simulink model "pmsm_with_saliency_and_damper"  (R2020a)
settings: Solver=FixedStepAuto  StartTime=0.0  StopTime=5  RelTol=1e-3  AbsTol=0.1
InitFcn:
  | vm=400;
  | wbase=314;
  | f=50;
  | xls=0.00291*wbase;
  | rs=0.037;
  | xmq=0.00324*wbase;
  | xmd=0.00324*wbase;
  | rkq=0.00144;
  | xlkq=0.6578;
  | rkd=0.1080;
  | xlkd=0.06577;
  | xaq=((1/xmq)+(1/xls)+(1/xlkq))^-1;
  | xad=((1/xmd)+(1/xls)+(1/xlkd))^-1;
  | Tl=50;
  | lamda_magnet=0.162;
  | p=10;
  | b=5*10^-3;
  | j=0.0003;
model workspace (MAT data in the model file):
  wb = Simulink.Parameter
  wb.DataType = 'auto'
  wb.Dimensions = [0 0]
settings Model: SnapshotBufferSize=100  SnapshotInterval=100  Creator=moham  LastModifiedBy=moham
settings SolverCC: ZeroCrossControl=EnableAll  AlgebraicLoopSolver=LineSearch
settings OptimizationCC: OptimizeBlockIOStorage=off  OptimizeDataStoreBuffers=off  BusAssignmentInplaceUpdate=off
settings DebuggingCC: SFUnexpectedBacktrackingDiag=warning  SFNoUnconditionalDefaultTransitionDiag=warning
settings RTWCC: Description=Generic Real-Time Target  GenCodeOnly=on  GenerateReport=on  BuildConfiguration=Debug  LaunchReport=on  RTWCompilerOptimization=on
settings CodeAppCC: ForceParamTrailComments=on  MaxIdLength=95  MATLABSourceComments=on  EnableCustomComments=on
settings GRTTargetCC: CombineSignalStateStructs=on  SupportVariableSizeSignals=on  MultiInstanceErrorCode=Warning

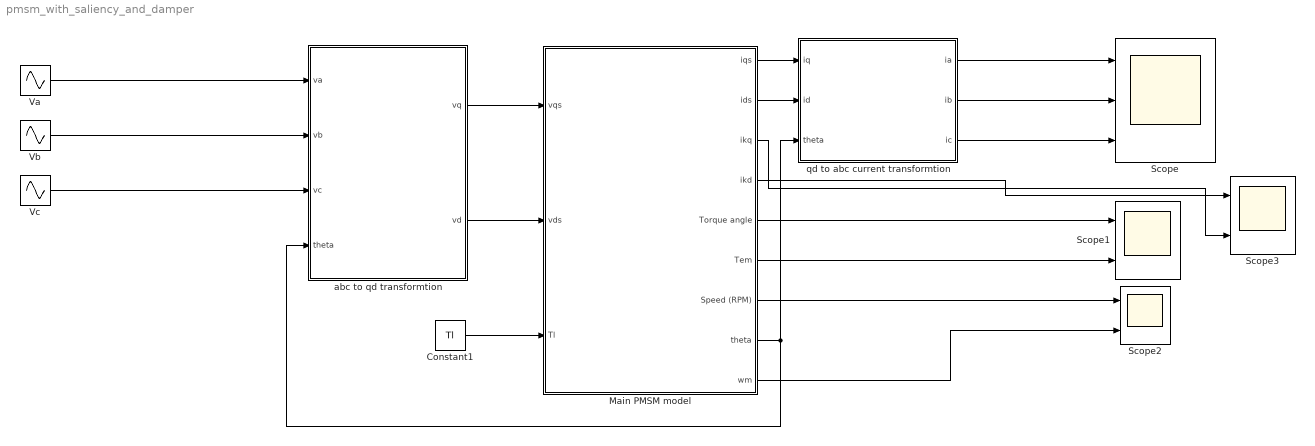
== system pmsm_with_saliency_and_damper ==
  Constant1 : Constant  Value=Tl
  Main PMSM model : Subsystem
  Scope : Scope  NumInputPorts=3
  Scope1 : Scope  NumInputPorts=2
  Scope2 : Scope  NumInputPorts=2
  Scope3 : Scope  NumInputPorts=2
  Va : Sin  Amplitude=vm  Frequency=2*pi*f  SampleTime=0.0001
  Vb : Sin  Amplitude=vm  Frequency=2*pi*f  Phase=-(2*pi/3)  SampleTime=0.0001
  Vc : Sin  Amplitude=vm  Frequency=2*pi*f  Phase=2*pi/3  SampleTime=0.0001
  abc to qd transformtion : Subsystem
  qd to abc current transformtion : Subsystem
  wires:
  Main PMSM model/2(ids) -> qd to abc current transformtion/2(id)
  Main PMSM model/8("theta ") -> abc to qd transformtion/4(theta), qd to abc current transformtion/3(theta)
  abc to qd transformtion/2(vd) -> Main PMSM model/2(vds)
  Constant1/1 -> Main PMSM model/3(Tl)
  abc to qd transformtion/1(vq) -> Main PMSM model/1(vqs)
  Main PMSM model/1(iqs) -> qd to abc current transformtion/1(iq)
  Va/1 -> abc to qd transformtion/1(va)
  Vb/1 -> abc to qd transformtion/2(vb)
  Vc/1 -> abc to qd transformtion/3(vc)
  qd to abc current transformtion/1(ia) -> Scope/1
  qd to abc current transformtion/2(ib) -> Scope/2
  qd to abc current transformtion/3(ic) -> Scope/3
  Main PMSM model/5(Torque angle) -> Scope1/1
  Main PMSM model/6(Tem) -> Scope1/2
  Main PMSM model/7(Speed (RPM)) -> Scope2/1
  Main PMSM model/9(wm) -> Scope2/2
  Main PMSM model/4(ikd) -> Scope3/1
  Main PMSM model/3(ikq) -> Scope3/2

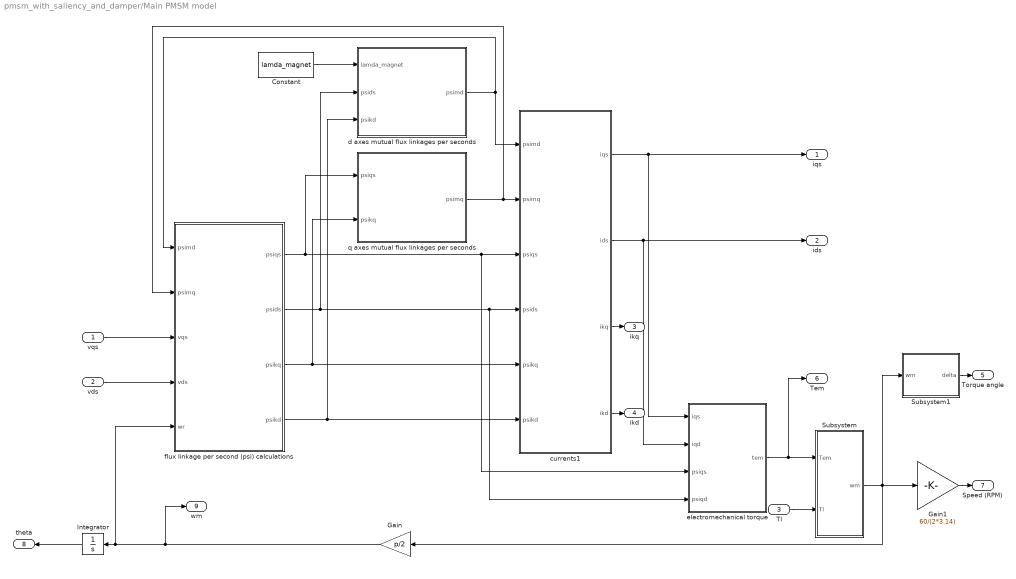
== system pmsm_with_saliency_and_damper/Main PMSM model ==
  vqs : Inport
  vds : Inport  Port=2
  Tl : Inport  Port=3
  Constant : Constant  Value=lamda_magnet
  Gain : Gain  Gain=p/2
  Gain1 : Gain  Gain=60/(2*3.14)
  Integrator : Integrator
  Subsystem : Subsystem
  Subsystem1 : Subsystem
  currents1 : Subsystem
  d axes mutual flux linkages per seconds : Subsystem
  electromechanical torque : Subsystem
  flux linkage per second (psi) calculations : Subsystem
  q axes mutual flux linkages per seconds : Subsystem
  iqs : Outport
  ids : Outport  Port=2
  ikq : Outport  Port=3
  ikd : Outport  Port=4
  Torque angle : Outport  Port=5
  Tem : Outport  Port=6
  Speed (RPM) : Outport  Port=7
  "theta " : Outport  Port=8
  wm : Outport  Port=9
  wires:
  currents1/2(ids) -> ids/1, electromechanical torque/2(iqd)
  q axes mutual flux linkages per seconds/1(psimq) -> flux linkage per second (psi) calculations/2(psimq), currents1/2(psimq)
  flux linkage per second (psi) calculations/2(psids) -> d axes mutual flux linkages per seconds/2(psids), currents1/4(psids), electromechanical torque/4(psiqd)
  electromechanical torque/1(tem) -> Tem/1, Subsystem/1(Tem)
  d axes mutual flux linkages per seconds/1(psimd) -> flux linkage per second (psi) calculations/1(psimd), currents1/1(psimd)
  currents1/1(iqs) -> iqs/1, electromechanical torque/1(iqs)
  currents1/4(ikd) -> ikd/1
  currents1/3(ikq) -> ikq/1
  Gain/1 -> wm/1, flux linkage per second (psi) calculations/5(wr), Integrator/1
  Constant/1 -> d axes mutual flux linkages per seconds/1(lamda_magnet)
  Subsystem/1(wm) -> Gain/1, Gain1/1, Subsystem1/1(wm)
  flux linkage per second (psi) calculations/3(psikq) -> q axes mutual flux linkages per seconds/2(psikq), currents1/5(psikq)
  flux linkage per second (psi) calculations/4(psikd) -> d axes mutual flux linkages per seconds/3(psikd), currents1/6(psikd)
  flux linkage per second (psi) calculations/1(psiqs) -> q axes mutual flux linkages per seconds/1(psiqs), currents1/3(psiqs), electromechanical torque/3(psiqs)
  vqs/1 -> flux linkage per second (psi) calculations/3(vqs)
  Gain1/1 -> Speed (RPM)/1
  vds/1 -> flux linkage per second (psi) calculations/4(vds)
  Subsystem1/1(delta) -> Torque angle/1
  Tl/1 -> Subsystem/2(Tl)
  Integrator/1 -> "theta "/1

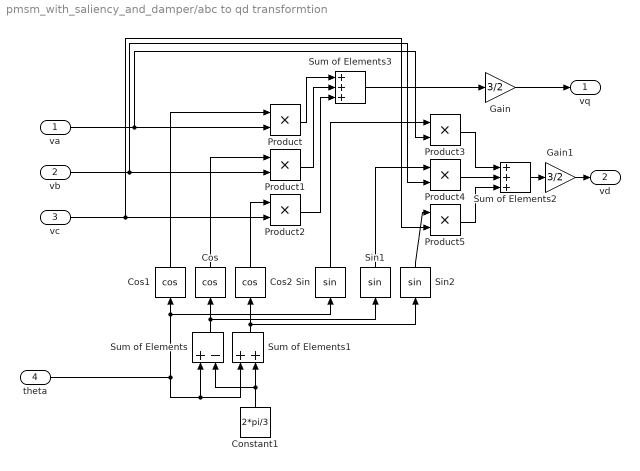
== system pmsm_with_saliency_and_damper/abc to qd transformtion ==
  va : Inport
  vb : Inport  Port=2
  vc : Inport  Port=3
  theta : Inport  Port=4
  Constant1 : Constant  Value=2*pi/3
  Cos : Trigonometry  Operator=cos
  Cos1 : Trigonometry  Operator=cos
  Cos2 : Trigonometry  Operator=cos
  Gain : Gain  Gain=3/2
  Gain1 : Gain  Gain=3/2
  Product{,1..5} (6 alike) : Product
  Sin : Trigonometry
  Sin1 : Trigonometry
  Sin2 : Trigonometry
  Sum of Elements : Sum  Inputs=+-
  Sum of Elements1 : Sum
  Sum of Elements2 : Sum  Inputs=+++
  Sum of Elements3 : Sum  Inputs=+++
  vq : Outport
  vd : Outport  Port=2
  wires:
  vc/1 -> Product2/2, Product5/2
  theta/1 -> Sum of Elements1/1, Sum of Elements/1, Sin/1, Cos1/1
  va/1 -> Product3/2, Product/2
  vb/1 -> Product1/2, Product4/2
  Cos/1 -> Product1/1
  Constant1/1 -> Sum of Elements1/2, Sum of Elements/2
  Cos1/1 -> Product/1
  Product/1 -> Sum of Elements3/1
  Sin/1 -> Product3/1
  Product1/1 -> Sum of Elements3/2
  Sum of Elements/1 -> Sin1/1, Cos/1
  Sin2/1 -> Product5/1
  Product5/1 -> Sum of Elements2/3
  Sum of Elements3/1 -> Gain/1
  Sum of Elements1/1 -> Sin2/1, Cos2/1
  Product3/1 -> Sum of Elements2/1
  Product4/1 -> Sum of Elements2/2
  Product2/1 -> Sum of Elements3/3
  Cos2/1 -> Product2/1
  Sin1/1 -> Product4/1
  Gain/1 -> vq/1
  Gain1/1 -> vd/1
  Sum of Elements2/1 -> Gain1/1

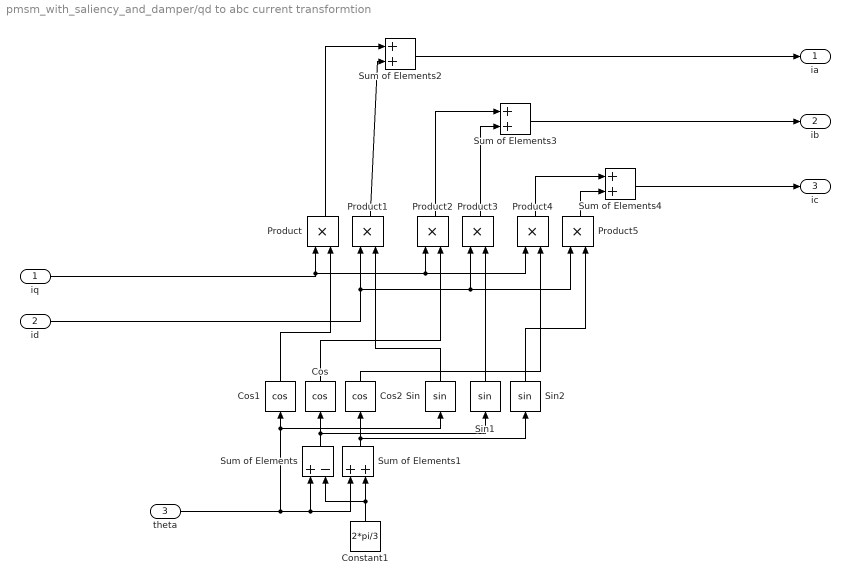
== system pmsm_with_saliency_and_damper/qd to abc current transformtion ==
  iq : Inport
  id : Inport  Port=2
  theta : Inport  Port=3
  Constant1 : Constant  Value=2*pi/3
  Cos : Trigonometry  Operator=cos
  Cos1 : Trigonometry  Operator=cos
  Cos2 : Trigonometry  Operator=cos
  Product{,1..5} (6 alike) : Product
  Sin : Trigonometry
  Sin1 : Trigonometry
  Sin2 : Trigonometry
  Sum of Elements : Sum  Inputs=+-
  Sum of Elements{1..4} (4 alike) : Sum
  ia : Outport
  ib : Outport  Port=2
  ic : Outport  Port=3
  wires:
  theta/1 -> Sin/1, Cos1/1, Sum of Elements1/1, Sum of Elements/1
  Constant1/1 -> Sum of Elements1/2, Sum of Elements/2
  Sum of Elements/1 -> Sin1/1, Cos/1
  Sum of Elements1/1 -> Sin2/1, Cos2/1
  iq/1 -> Product2/1, Product4/1, Product/1
  Cos1/1 -> Product/2
  id/1 -> Product1/1, Product3/1, Product5/1
  Sin/1 -> Product1/2
  Cos/1 -> Product2/2
  Sin1/1 -> Product3/2
  Cos2/1 -> Product4/2
  Sin2/1 -> Product5/2
  Product1/1 -> Sum of Elements2/2
  Product/1 -> Sum of Elements2/1
  Product3/1 -> Sum of Elements3/2
  Product2/1 -> Sum of Elements3/1
  Product5/1 -> Sum of Elements4/2
  Product4/1 -> Sum of Elements4/1
  Sum of Elements2/1 -> ia/1
  Sum of Elements3/1 -> ib/1
  Sum of Elements4/1 -> ic/1

== system pmsm_with_saliency_and_damper/Main PMSM model/Subsystem ==
  Tem : Inport
  Tl : Inport  Port=2
  Constant2 : Constant  Value=b
  Constant3 : Constant  Value=j
  Divide : Product  Inputs=*/
  Integrator1 : Integrator
  Product2 : Product
  Sum of Elements1 : Sum  Inputs=+--
  wm : Outport
  wires:
  Tem/1 -> Sum of Elements1/1
  Sum of Elements1/1 -> Divide/1
  Constant3/1 -> Divide/2
  Product2/1 -> Sum of Elements1/3
  Divide/1 -> Integrator1/1
  Integrator1/1 -> wm/1, Product2/1
  Tl/1 -> Sum of Elements1/2
  Constant2/1 -> Product2/2

== system pmsm_with_saliency_and_damper/Main PMSM model/Subsystem1 ==
  wm : Inport
  Constant : Constant  Value=p/2
  Constant2 : Constant  Value=2*pi*f
  Integrator1 : Integrator
  Product : Product
  Sum of Elements : Sum  Inputs=+-
  delta : Outport
  wires:
  Sum of Elements/1 -> Integrator1/1
  Integrator1/1 -> delta/1
  Constant2/1 -> Sum of Elements/1
  wm/1 -> Product/1
  Product/1 -> Sum of Elements/2
  Constant/1 -> Product/2

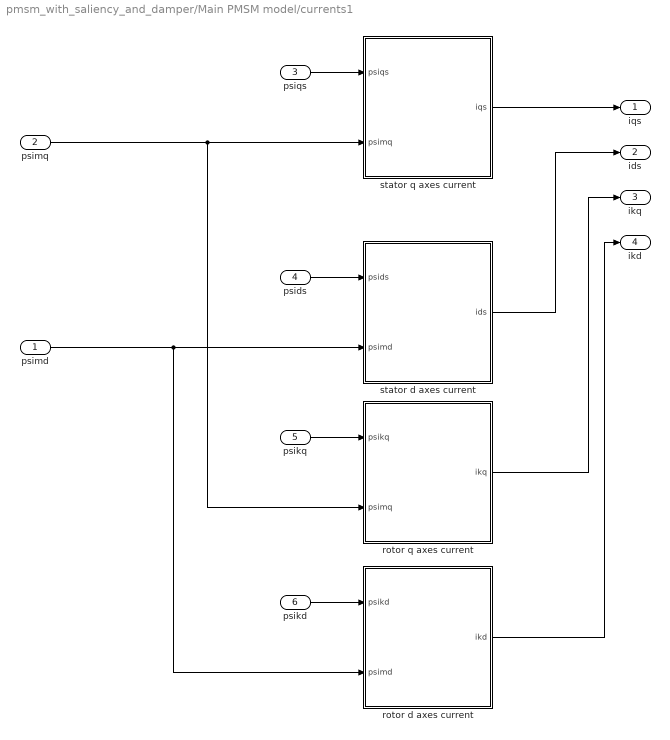
== system pmsm_with_saliency_and_damper/Main PMSM model/currents1 ==
  psimd : Inport
  psimq : Inport  Port=2
  psiqs : Inport  Port=3
  psids : Inport  Port=4
  psikq : Inport  Port=5
  psikd : Inport  Port=6
  rotor d axes current : Subsystem
  rotor q axes current : Subsystem
  stator d axes current : Subsystem
  stator q axes current : Subsystem
  iqs : Outport
  ids : Outport  Port=2
  ikq : Outport  Port=3
  ikd : Outport  Port=4
  wires:
  rotor q axes current/1(ikq) -> ikq/1
  stator q axes current/1(iqs) -> iqs/1
  psikd/1 -> rotor d axes current/1(psikd)
  psids/1 -> stator d axes current/1(psids)
  psimd/1 -> rotor d axes current/2(psimd), stator d axes current/2(psimd)
  stator d axes current/1(ids) -> ids/1
  psimq/1 -> stator q axes current/2(psimq), rotor q axes current/2(psimq)
  rotor d axes current/1(ikd) -> ikd/1
  psikq/1 -> rotor q axes current/1(psikq)
  psiqs/1 -> stator q axes current/1(psiqs)

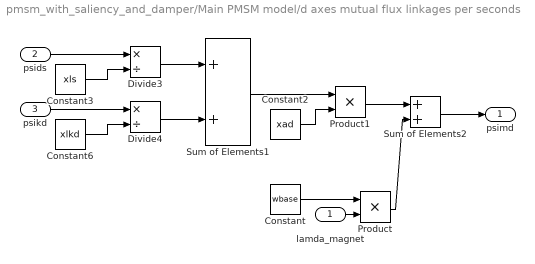
== system pmsm_with_saliency_and_damper/Main PMSM model/d axes mutual flux linkages per seconds ==
  lamda_magnet : Inport
  psids : Inport  Port=2
  psikd : Inport  Port=3
  Constant : Constant  Value=wbase
  Constant2 : Constant  Value=xad
  Constant3 : Constant  Value=xls
  Constant6 : Constant  Value=xlkd
  Divide3 : Product  Inputs=*/
  Divide4 : Product  Inputs=*/
  Product : Product
  Product1 : Product
  Sum of Elements1 : Sum
  Sum of Elements2 : Sum
  psimd : Outport
  wires:
  lamda_magnet/1 -> Product/2
  Sum of Elements1/1 -> Product1/1
  Constant/1 -> Product/1
  Product1/1 -> Sum of Elements2/1
  Constant2/1 -> Product1/2
  Sum of Elements2/1 -> psimd/1
  Product/1 -> Sum of Elements2/2
  psids/1 -> Divide3/1
  psikd/1 -> Divide4/1
  Constant3/1 -> Divide3/2
  Constant6/1 -> Divide4/2
  Divide3/1 -> Sum of Elements1/1
  Divide4/1 -> Sum of Elements1/2

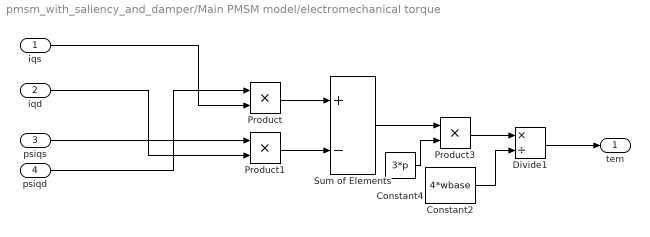
== system pmsm_with_saliency_and_damper/Main PMSM model/electromechanical torque ==
  iqs : Inport
  iqd : Inport  Port=2
  psiqs : Inport  Port=3
  psiqd : Inport  Port=4
  Constant2 : Constant  Value=4*wbase
  Constant4 : Constant  Value=3*p
  Divide1 : Product  Inputs=*/
  Product : Product
  Product1 : Product
  Product3 : Product
  Sum of Elements : Sum  Inputs=+-
  tem : Outport
  wires:
  iqs/1 -> Product/2
  Product1/1 -> Sum of Elements/2
  Product/1 -> Sum of Elements/1
  Sum of Elements/1 -> Product3/1
  psiqs/1 -> Product1/1
  psiqd/1 -> Product/1
  iqd/1 -> Product1/2
  Constant4/1 -> Product3/2
  Constant2/1 -> Divide1/2
  Product3/1 -> Divide1/1
  Divide1/1 -> tem/1

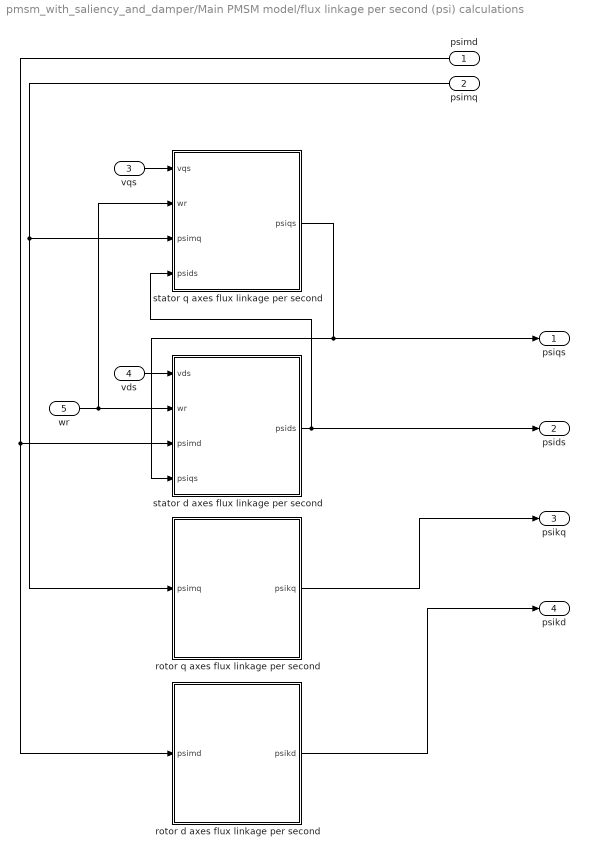
== system pmsm_with_saliency_and_damper/Main PMSM model/flux linkage per second (psi) calculations ==
  psimd : Inport
  psimq : Inport  Port=2
  vqs : Inport  Port=3
  vds : Inport  Port=4
  wr : Inport  Port=5
  rotor d axes flux linkage per second : Subsystem
  rotor q axes flux linkage per second : Subsystem
  stator d axes flux linkage per second : Subsystem
  stator q axes flux linkage per second : Subsystem
  psiqs : Outport
  psids : Outport  Port=2
  psikq : Outport  Port=3
  psikd : Outport  Port=4
  wires:
  stator q axes flux linkage per second/1(psiqs) -> psiqs/1, stator d axes flux linkage per second/4(psiqs)
  rotor q axes flux linkage per second/1(psikq) -> psikq/1
  wr/1 -> stator q axes flux linkage per second/2(wr), stator d axes flux linkage per second/2(wr)
  stator d axes flux linkage per second/1(psids) -> psids/1, stator q axes flux linkage per second/4(psids)
  psimq/1 -> stator q axes flux linkage per second/3(psimq), rotor q axes flux linkage per second/1(psimq)
  vqs/1 -> stator q axes flux linkage per second/1(vqs)
  rotor d axes flux linkage per second/1(psikd) -> psikd/1
  psimd/1 -> rotor d axes flux linkage per second/1(psimd), stator d axes flux linkage per second/3(psimd)
  vds/1 -> stator d axes flux linkage per second/1(vds)

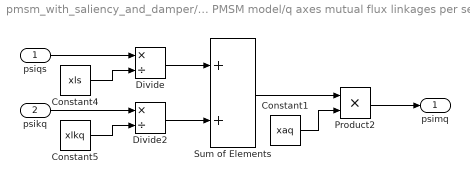
== system pmsm_with_saliency_and_damper/Main PMSM model/q axes mutual flux linkages per seconds ==
  psiqs : Inport
  psikq : Inport  Port=2
  Constant1 : Constant  Value=xaq
  Constant4 : Constant  Value=xls
  Constant5 : Constant  Value=xlkq
  Divide : Product  Inputs=*/
  Divide2 : Product  Inputs=*/
  Product2 : Product
  Sum of Elements : Sum
  psimq : Outport
  wires:
  Divide2/1 -> Sum of Elements/2
  Constant1/1 -> Product2/2
  Constant5/1 -> Divide2/2
  psikq/1 -> Divide2/1
  psiqs/1 -> Divide/1
  Divide/1 -> Sum of Elements/1
  Product2/1 -> psimq/1
  Sum of Elements/1 -> Product2/1
  Constant4/1 -> Divide/2

== system pmsm_with_saliency_and_damper/Main PMSM model/currents1/rotor d axes current ==
  psikd : Inport
  psimd : Inport  Port=2
  Constant : Constant  Value=xlkd
  Divide : Product  Inputs=*/
  Sum of Elements : Sum  Inputs=+-
  ikd : Outport
  wires:
  Divide/1 -> ikd/1
  Constant/1 -> Divide/2
  Sum of Elements/1 -> Divide/1
  psimd/1 -> Sum of Elements/2
  psikd/1 -> Sum of Elements/1

== system pmsm_with_saliency_and_damper/Main PMSM model/currents1/rotor q axes current ==
  psikq : Inport
  psimq : Inport  Port=2
  Constant : Constant  Value=xlkq
  Divide : Product  Inputs=*/
  Sum of Elements : Sum  Inputs=+-
  ikq : Outport
  wires:
  Divide/1 -> ikq/1
  Constant/1 -> Divide/2
  Sum of Elements/1 -> Divide/1
  psimq/1 -> Sum of Elements/2
  psikq/1 -> Sum of Elements/1

== system pmsm_with_saliency_and_damper/Main PMSM model/currents1/stator d axes current ==
  psids : Inport
  psimd : Inport  Port=2
  Constant : Constant  Value=xls
  Divide : Product  Inputs=*/
  Sum of Elements : Sum  Inputs=+-
  ids : Outport
  wires:
  Divide/1 -> ids/1
  Constant/1 -> Divide/2
  Sum of Elements/1 -> Divide/1
  psimd/1 -> Sum of Elements/2
  psids/1 -> Sum of Elements/1

== system pmsm_with_saliency_and_damper/Main PMSM model/currents1/stator q axes current ==
  psiqs : Inport
  psimq : Inport  Port=2
  Constant : Constant  Value=xls
  Divide : Product  Inputs=*/
  Sum of Elements : Sum  Inputs=+-
  iqs : Outport
  wires:
  Divide/1 -> iqs/1
  Constant/1 -> Divide/2
  Sum of Elements/1 -> Divide/1
  psimq/1 -> Sum of Elements/2
  psiqs/1 -> Sum of Elements/1

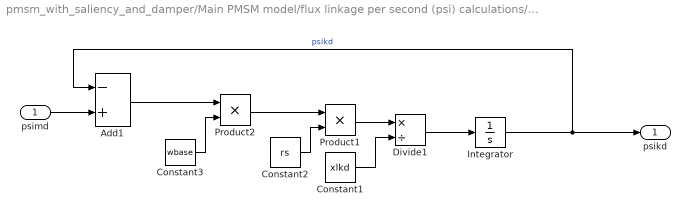
== system pmsm_with_saliency_and_damper/Main PMSM model/flux linkage per second (psi) calculations/rotor d axes flux linkage per second ==
  psimd : Inport
  Add1 : Sum  Inputs=-+
  Constant1 : Constant  Value=xlkd
  Constant2 : Constant  Value=rs
  Constant3 : Constant  Value=wbase
  Divide1 : Product  Inputs=*/
  Integrator : Integrator
  Product1 : Product
  Product2 : Product
  psikd : Outport
  wires:
  psimd/1 -> Add1/2
  Integrator/1 -> psikd/1, Add1/1  "psikd"
  Add1/1 -> Product2/1
  Product2/1 -> Product1/1
  Constant2/1 -> Product1/2
  Product1/1 -> Divide1/1
  Constant3/1 -> Product2/2
  Divide1/1 -> Integrator/1
  Constant1/1 -> Divide1/2

== system pmsm_with_saliency_and_damper/Main PMSM model/flux linkage per second (psi) calculations/rotor q axes flux linkage per second ==
  psimq : Inport
  Add1 : Sum  Inputs=-+
  Constant1 : Constant  Value=xlkq
  Constant2 : Constant  Value=rs
  Constant3 : Constant  Value=wbase
  Divide1 : Product  Inputs=*/
  Integrator : Integrator
  Product1 : Product
  Product2 : Product
  psikq : Outport
  wires:
  psimq/1 -> Add1/2
  Divide1/1 -> Integrator/1
  Integrator/1 -> Add1/1, psikq/1  "psikq"
  Add1/1 -> Product2/1
  Constant1/1 -> Divide1/2
  Product1/1 -> Divide1/1
  Constant2/1 -> Product1/2
  Product2/1 -> Product1/1
  Constant3/1 -> Product2/2

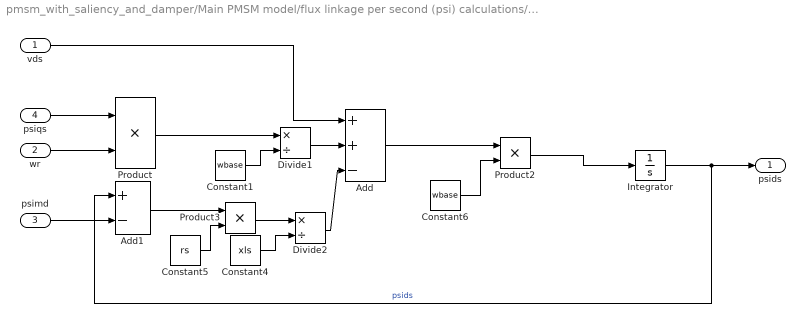
== system pmsm_with_saliency_and_damper/Main PMSM model/flux linkage per second (psi) calculations/stator d axes flux linkage per second ==
  vds : Inport
  wr : Inport  Port=2
  psimd : Inport  Port=3
  psiqs : Inport  Port=4
  Add : Sum  Inputs=++-
  Add1 : Sum  Inputs=+-
  Constant1 : Constant  Value=wbase
  Constant4 : Constant  Value=xls
  Constant5 : Constant  Value=rs
  Constant6 : Constant  Value=wbase
  Divide1 : Product  Inputs=*/
  Divide2 : Product  Inputs=*/
  Integrator : Integrator
  Product : Product
  Product2 : Product
  Product3 : Product
  psids : Outport
  wires:
  psimd/1 -> Add1/2
  vds/1 -> Add/1
  Integrator/1 -> psids/1, Add1/1  "psids"
  psiqs/1 -> Product/1
  wr/1 -> Product/2
  Add/1 -> Product2/1
  Divide1/1 -> Add/2
  Constant5/1 -> Product3/2
  Constant4/1 -> Divide2/2
  Add1/1 -> Product3/1
  Divide2/1 -> Add/3
  Product3/1 -> Divide2/1
  Constant1/1 -> Divide1/2
  Product/1 -> Divide1/1
  Constant6/1 -> Product2/2
  Product2/1 -> Integrator/1

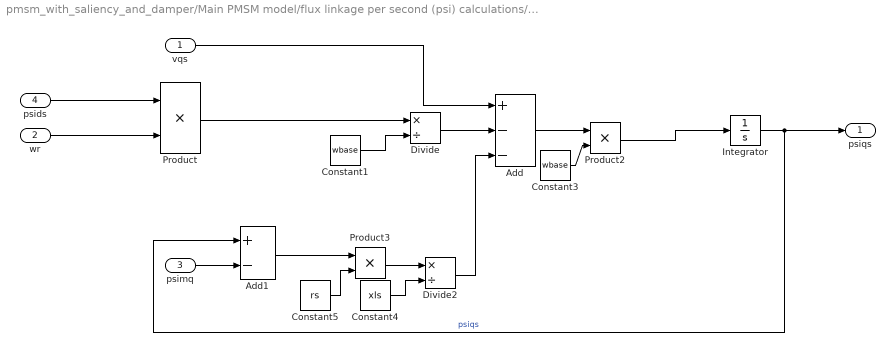
== system pmsm_with_saliency_and_damper/Main PMSM model/flux linkage per second (psi) calculations/stator q axes flux linkage per second ==
  vqs : Inport
  wr : Inport  Port=2
  psimq : Inport  Port=3
  psids : Inport  Port=4
  Add : Sum  Inputs=+--
  Add1 : Sum  Inputs=+-
  Constant1 : Constant  Value=wbase
  Constant3 : Constant  Value=wbase
  Constant4 : Constant  Value=xls
  Constant5 : Constant  Value=rs
  Divide : Product  Inputs=*/
  Divide2 : Product  Inputs=*/
  Integrator : Integrator
  Product : Product
  Product2 : Product
  Product3 : Product
  psiqs : Outport
  wires:
  psimq/1 -> Add1/2
  vqs/1 -> Add/1
  Integrator/1 -> psiqs/1, Add1/1  "psiqs"
  psids/1 -> Product/1
  Add/1 -> Product2/1
  wr/1 -> Product/2
  Divide/1 -> Add/2
  Product/1 -> Divide/1
  Constant1/1 -> Divide/2
  Constant3/1 -> Product2/2
  Product2/1 -> Integrator/1
  Constant5/1 -> Product3/2
  Add1/1 -> Product3/1
  Divide2/1 -> Add/3
  Constant4/1 -> Divide2/2
  Product3/1 -> Divide2/1
